simulink model "sampleModel374"  (R2021b)
settings: Solver=VariableStepAuto  StartTime=0.0  StopTime=10.0  RelTol=1e-3
undefined symbols (not defined in the file or in its folder): Newton, Raphson
libraries: simulink x1
settings Model: Creator=user  LastModifiedBy=user

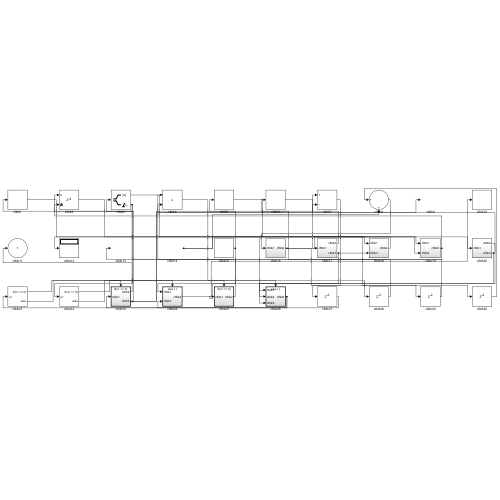
[thumbnail: Simulink's stored preview of the top-level diagram]
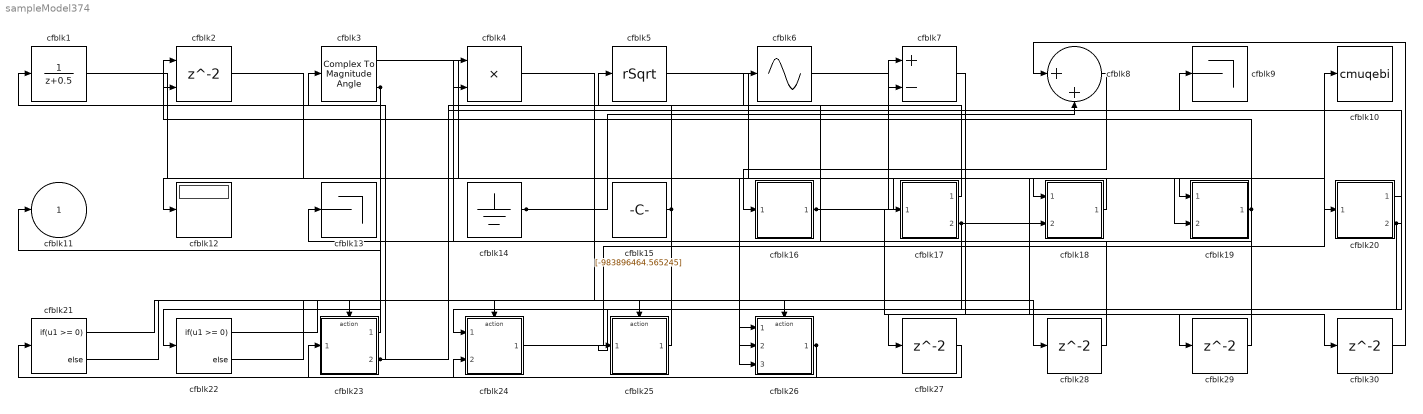
== system sampleModel374 ==
  cfblk1 : DiscreteTransferFcn  SampleTime=1
  cfblk10 : ToWorkspace  VariableName=cmuqebi  SaveFormat=Timeseries  SampleTime=-1
  cfblk12 : Display
  cfblk13 : Terminator
  cfblk14 : Ground
  cfblk15 : Constant  Value=[-983896464.565245]  SampleTime=1
  cfblk16 : Subsystem
  cfblk17 : Subsystem
  cfblk18 : Subsystem
  cfblk19 : Subsystem
  cfblk2 : Delay  ShowEnablePort=on  SampleTime=1
      settings: InputPortMap=u0,e6
  cfblk20 : Subsystem
  cfblk21 : If  IfExpression=u1 >= 0  SampleTime=1
  cfblk22 : If  IfExpression=u1 >= 0  SampleTime=1
  cfblk23 : Subsystem  TreatAsAtomicUnit=on
  cfblk24 : Subsystem  TreatAsAtomicUnit=on
  cfblk25 : Subsystem  TreatAsAtomicUnit=on
  cfblk26 : Subsystem  TreatAsAtomicUnit=on
  cfblk{27..30} (4 alike) : Delay  SampleTime=1
  cfblk3 : ComplexToMagnitudeAngle
  cfblk4 : Product  Inputs=**
  cfblk5 : Sqrt  Operator=rSqrt  AlgorithmType=Newton-Raphson  SaturateOnIntegerOverflow=on
  cfblk6 : Sin  TimeSource=Use external signal  SampleTime=0
  cfblk7 : Sum  Inputs=+-
  cfblk8 : Sum  Inputs=|++
  cfblk9 : Terminator
  cfblk11 : Outport
  wires:
  cfblk16/1(cfblk2) -> cfblk18/1(cfblk1), cfblk30/1
  cfblk8/1 -> cfblk16/1(cfblk1)
  cfblk19/1(cfblk2) -> cfblk13/1, cfblk2/2
  cfblk17/1(cfblk2) -> cfblk7/1
  cfblk24/1(cfblk2) -> cfblk10/1
  cfblk14/1 -> cfblk19/1(cfblk1), cfblk8/2
  cfblk5/1 -> cfblk20/1(cfblk1)
  cfblk2/1 -> cfblk18/2(cfblk3)
  cfblk20/1(cfblk2) -> cfblk25/1(cfblk1)
  cfblk3/1 -> cfblk19/2(cfblk4)
  cfblk3/2 -> cfblk1/1, cfblk22/1
  cfblk18/1(cfblk2) -> cfblk12/1
  cfblk23/1(cfblk2) -> cfblk11/1
  cfblk23/2(cfblk5) -> cfblk2/1, cfblk9/1, cfblk7/2
  cfblk6/1 -> cfblk17/1(cfblk1)
  cfblk1/1 -> cfblk26/1(cfblk1)
  cfblk26/1(cfblk2) -> cfblk21/1, cfblk24/2(cfblk3)
  cfblk20/2(cfblk4) -> cfblk4/1, cfblk26/2(cfblk4)
  cfblk15/1 -> cfblk24/1(cfblk1), cfblk5/1
  cfblk25/1(cfblk2) -> cfblk4/2
  cfblk17/2(cfblk3) -> cfblk26/3(cfblk5), cfblk29/1
  cfblk21/1 -> cfblk23/Action
  cfblk21/2 -> cfblk24/Action
  cfblk22/1 -> cfblk25/Action
  cfblk22/2 -> cfblk26/Action
  cfblk7/1 -> cfblk27/1
  cfblk27/1 -> cfblk23/1(cfblk1)
  cfblk4/1 -> cfblk28/1
  cfblk28/1 -> cfblk3/1
  cfblk29/1 -> cfblk6/1
  cfblk30/1 -> cfblk8/1

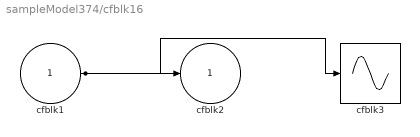
== system sampleModel374/cfblk16 ==
  cfblk1 : Inport
  cfblk3 : Sin  TimeSource=Use external signal  SampleTime=0
  cfblk2 : Outport
  wires:
  cfblk1/1 -> cfblk2/1, cfblk3/1

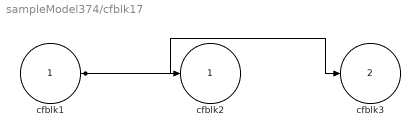
== system sampleModel374/cfblk17 ==
  cfblk1 : Inport
  cfblk2 : Outport
  cfblk3 : Outport  Port=2
  wires:
  cfblk1/1 -> cfblk3/1, cfblk2/1

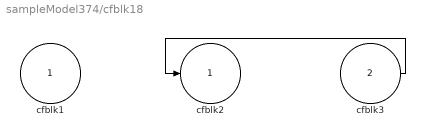
== system sampleModel374/cfblk18 ==
  cfblk1 : Inport
  cfblk3 : Inport  Port=2
  cfblk2 : Outport
  wires:
  cfblk3/1 -> cfblk2/1

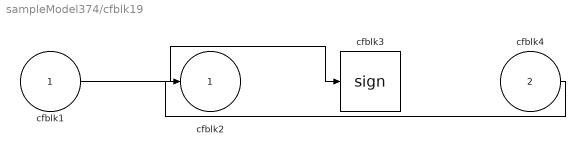
== system sampleModel374/cfblk19 ==
  cfblk1 : Inport
  cfblk4 : Inport  Port=2
  cfblk3 : Signum
  cfblk2 : Outport
  wires:
  cfblk1/1 -> cfblk3/1
  cfblk4/1 -> cfblk2/1

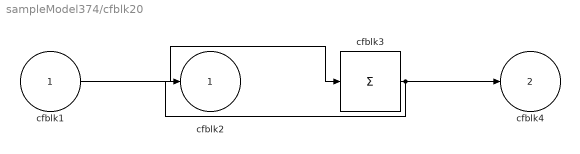
== system sampleModel374/cfblk20 ==
  cfblk1 : Inport
  cfblk3 : Sum  Inputs=+
  cfblk2 : Outport
  cfblk4 : Outport  Port=2
  wires:
  cfblk1/1 -> cfblk3/1
  cfblk3/1 -> cfblk2/1, cfblk4/1

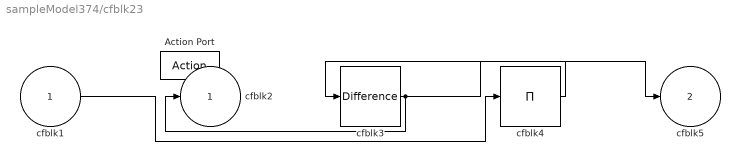
== system sampleModel374/cfblk23 ==
  cfblk1 : Inport
  Action Port : ActionPort  ActionPortLabel=if(u1 >= 0)
  cfblk3 : simulink/Discrete/Difference  ICPrevInput=0.0  OutMin=[]  OutMax=[]  OutDataTypeStr=Inherit: Inherit via back propagation  OutDataType=fixdt(1, 16)  OutScaling=2^-10  DoSatur=off
  cfblk4 : Product  Inputs=*
  cfblk2 : Outport
  cfblk5 : Outport  Port=2
  wires:
  cfblk4/1 -> cfblk3/1
  cfblk3/1 -> cfblk2/1, cfblk5/1
  cfblk1/1 -> cfblk4/1

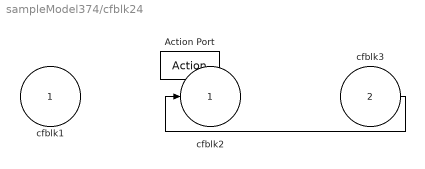
== system sampleModel374/cfblk24 ==
  cfblk1 : Inport
  cfblk3 : Inport  Port=2
  Action Port : ActionPort  ActionPortLabel=else
  cfblk2 : Outport
  wires:
  cfblk3/1 -> cfblk2/1

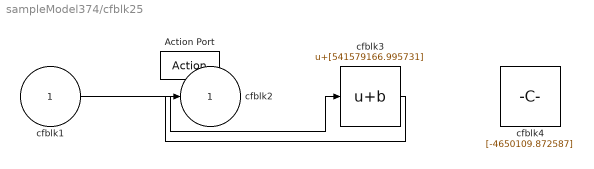
== system sampleModel374/cfblk25 ==
  cfblk1 : Inport
  Action Port : ActionPort  ActionPortLabel=if(u1 >= 0)
  cfblk3 : Bias  Bias=[541579166.995731]
  cfblk4 : Constant  Value=[-4650109.872587]  SampleTime=1
  cfblk2 : Outport
  wires:
  cfblk1/1 -> cfblk3/1
  cfblk3/1 -> cfblk2/1

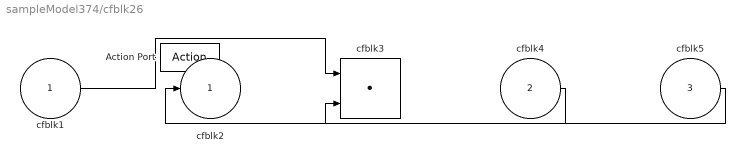
== system sampleModel374/cfblk26 ==
  cfblk1 : Inport
  cfblk4 : Inport  Port=2
  cfblk5 : Inport  Port=3
  Action Port : ActionPort  ActionPortLabel=else
  cfblk3 : DotProduct  InputSameDT=on  OutDataTypeStr=Inherit: Inherit via internal rule
  cfblk2 : Outport
  wires:
  cfblk5/1 -> cfblk2/1
  cfblk1/1 -> cfblk3/1
  cfblk4/1 -> cfblk3/2
